simulink model "scalar_quantizer_example2"  (Simulink 5.0)
settings: Solver=FixedStepDiscrete  SolverMode=SingleTasking  StartTime=0.0  StopTime=0.49  RelTol=1e-3
PreLoadFcn:
  | load mtlb;
undefined symbols (not defined in the file or in its folder): Mag, mtlb
libraries: dspsnks4 x5, dspquant2 x5, dsparch4 x4, dspsigops x2, dspsrcs4 x1, dspstat3 x1, dspxfrm3 x1, dspsolvers x1, dspbuff3 x1
settings Model: RequirementInfo=9  CovMetricSettings=d  Creator=dshpak  LastModifiedBy=cclarke  ExtModeTrigMode=oneshot  ExtModeArmWhenConnect=off  ExtModeAutoUpdateStatusClock=off  SaveTime=off  SaveOutput=off  SaveFormat=Structure  LimitDataPoints=off  IntegerOverflowMsg=none  BlockReductionOpt=off  BooleanDataType=off  ZeroCrossControl=UseLocalSettings  TargetHWChar=2  TargetHWWordLengths=8,16,32,32  RTWMathFcnLibMatFile=iso_c_tmw.mat  RTWOptions="-aEnforceIntegerDowncast=1 -aFoldNonRolledExpr=1 -aInlineInvariantSignals=0 -aInlineParameters=0 -aLocalBlockOutputs=1 -aRollThreshold=5 -aRTWVerbose=1 -aForceParamTrailComments=0 -aGenerateComments=1 -aIgnoreCustomStorageClasses=1 -aIncHierarchyInIds=0 -aMaxRTWIdLen=31 -aShowEliminatedStatements=1 -aReadOnly=0 -aTargetFcnLib=\"iso_c_tmw.mat\" -aIncDataTypeInIds=0 -aPrefixModelToSubsysFcnNames=1 -aInlinedPrmAccess=\"Literals\" -aGenerateFullHeader=1 -aIsPILTarget=0 -aGenerateReport=0 -aLogVarNameModifier=\"rt_\" -aExtMode=0 -aExtModeStaticAlloc=0 -aExtModeTesting=0 -aExtModeStaticAllocSize=1000000 -aExtModeTransport=0"

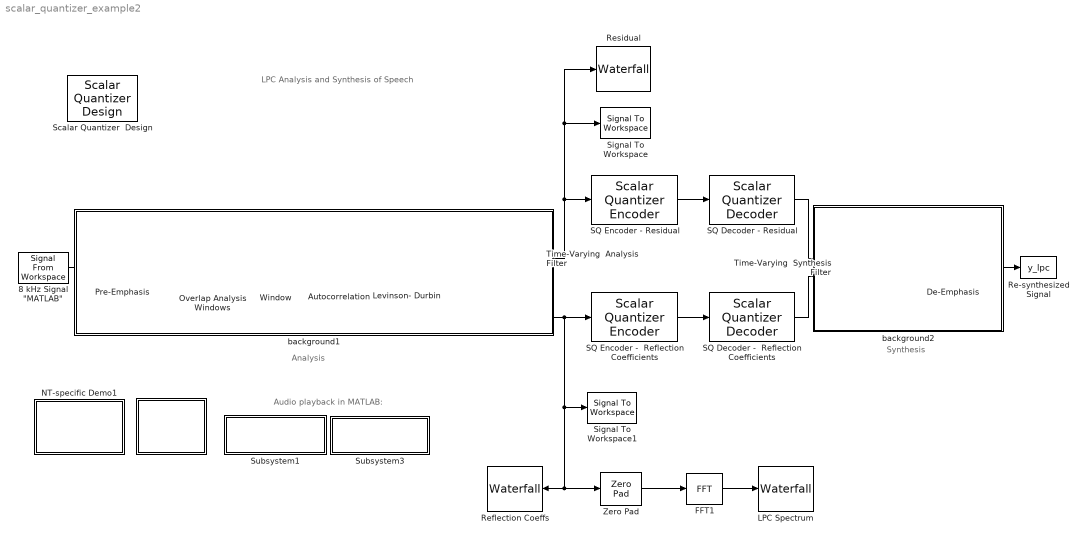
== system scalar_quantizer_example2 ==
  note: LPC Analysis and Synthesis of Speech
  note: Analysis
  note: Synthesis
  note: Audio playback in MATLAB:
  " " : Subsystem
      mask Type: Frame-Based Simulation Info
      mask Display: disp('Info')
  "8 kHz Signal \"MATLAB\"" : dspsrcs4/Signal From Workspace  X=mtlb*0.32  Ts=1/8000  nsamps=80  OutputAfterFinalValue=Setting to zero
  Autocorrelation : dspstat3/Autocorrelation  AllPositiveLags=off  maxlag=12  bias=Biased  domain=Time  roundingMode=Floor  overflowMode=off
  De-Emphasis : dsparch4/Digital Filter  TypePopup=IIR (all poles)  IIRFiltStruct=Direct form II transposed  AllPoleFiltStruct=Direct form  FIRFiltStruct=Direct form  CoeffSource=Specify via dialog  NumCoeffs=[1 -.95]  DenCoeffs=[1 -.95]  BiQuadCoeffs=[1 0.3 0.4 1 0.1 0.2]  LatticeCoeffs=[0.2 0.4]  denIgnore=on  FiltPerSampPopup=One filter per frame  IC=0  ICnum=0  ICden=0  roundingMode=Floor  overflowMode=off
  FFT1 : dspxfrm3/FFT  CompMethod=Table lookup  TableOpt=Speed  BitRevOrder=off  SkipNorm=off  roundingMode=Floor  overflowMode=off
  LPC Spectrum : dspsnks4/Waterfall  TraceProperties=off  NumTraces=10  CMapStr=autumn  TNewest=0.35  TOldest=0.1  HistoryLength=100  HistoryFull=Overwrite  UpdateInterval=1  ExportMode=All visible  MLExportName=ExportData  AutoExport=off  DisplayProperties=off  MouseMode=Orbit  AxisGrid=off  Snapshot=off  Suspend=off  SyncSnapshots=off  OpenScopeAtSimStart=off  FigPos=[452 44 407 353]  CameraView=[89945.9047576273 49093.2447020758 -7462.52930692949 -16.6995606364064 71 5.5 2.5389885178677 -5.30668596526891 0.808418434368868 0.0592442608385446 5.583225828012 14.2 1]  InportDimsHint=[129 1]  AxisProperties=off  AxisColor=[1 1 1]*.9  XLabel=Frequency  YLabel=Mag^2  ZLabel=History  TriggerProperties=off  TrigStartMode=Immediately  TrigStartT=10  TrigStartN=1000  TrigStartFcn=trigPower  TrigStopMode=Never  TrigStopT=0.1  TrigStopN=10  TrigStopFcn=trigend  TrigRearmMode=User-defined  TrigRearmT=0  TrigRearmN=100  TrigRearmFcn=trigrearm  XformProperties=off  XformMode=FFT->Mag dB Fs/2  XformFcn=fliplr  XformExpr=20*log10(abs(u(129:2:end)))
      settings: YMin=-44.6156897764664  YMax=11.2165685036536
  Levinson- Durbin : dspsolvers/Levinson-Durbin  coeffOutFcn=K  outP=off  zeroInpHandling=on
  NT-specific Demo1 : Subsystem
      settings: OpenFcn=dsplpc_win32
      mask Type: NT-only Demo
      mask Display: disp('PC/Windows\nLPC Demo')
  Overlap Analysis Windows : dspbuff3/Buffer  N=160  V=80  ic=0
  Pre-Emphasis : dsparch4/Digital Filter  TypePopup=FIR (all zeros)  IIRFiltStruct=Direct form II transposed  AllPoleFiltStruct=Direct form  FIRFiltStruct=Direct form  CoeffSource=Specify via dialog  NumCoeffs=[1 -.95]  DenCoeffs=[1 0.1]  BiQuadCoeffs=[1 0.3 0.4 1 0.1 0.2]  LatticeCoeffs=[0.2 0.4]  denIgnore=on  FiltPerSampPopup=One filter per frame  IC=0  ICnum=0  ICden=0  roundingMode=Floor  overflowMode=off
  Re-synthesized Signal : ToWorkspace  VariableName=y_lpc  SampleTime=-1  SaveFormat=Array
  Reflection Coeffs : dspsnks4/Waterfall  Orientation=left  TraceProperties=off  NumTraces=10  CMapStr=autumn  TNewest=0.7  TOldest=0.1  HistoryLength=50  HistoryFull=Overwrite  UpdateInterval=1  ExportMode=All visible  MLExportName=ExportData2  AutoExport=off  DisplayProperties=off  MouseMode=Orbit  AxisGrid=on  Snapshot=off  Suspend=off  SyncSnapshots=off  OpenScopeAtSimStart=off  FigPos=[35 41 410 358]  CameraView=[73343.0440471642 150383.489958622 -231607.055769344 -0.0735265549347769 7.5 5.5 0.547487828138618 -2.62241953831449 4.03911084299836 0.00240035045613671 1 7.88928028685195 5.25952019123463]  InportDimsHint=[12 1]  AxisProperties=off  AxisColor=[1 1 1]*.9  XLabel=Coefficient  YLabel=RC Amplitude  ZLabel=History  TriggerProperties=off  TrigStartMode=Immediately  TrigStartT=10  TrigStartN=1000  TrigStartFcn=trigPower  TrigStopMode=Never  TrigStopT=0.1  TrigStopN=10  TrigStopFcn=trigend  TrigRearmMode=User-defined  TrigRearmT=0  TrigRearmN=100  TrigRearmFcn=trigrearm  XformProperties=off  XformMode=None  XformFcn=fliplr  XformExpr=20*log10(abs(u(129:2:end)))
      settings: YMin=-1.02418361455266  YMax=0.877130504683106
  Residual : dspsnks4/Waterfall  TraceProperties=off  NumTraces=10  CMapStr=autumn  TNewest=0.7  TOldest=0.1  HistoryLength=50  HistoryFull=Overwrite  UpdateInterval=1  ExportMode=All visible  MLExportName=ExportData2  AutoExport=off  DisplayProperties=off  MouseMode=Orbit  AxisGrid=on  Snapshot=off  Suspend=off  SyncSnapshots=off  OpenScopeAtSimStart=off  FigPos=[524 276 410 358]  CameraView=[62164.2347969079 1792549.89917746 -405278.370332737 -0.097024155318337 44.5 5.5 0.575539043328793 -33.5051317778483 7.57548038023531 0.00104183380472551 1 92.0645761641202 10.3443344004629]  InportDimsHint=[80 1]  AxisProperties=off  AxisColor=[1 1 1]*.9  XLabel=Coefficient  YLabel=Amplitude  ZLabel=History  TriggerProperties=off  TrigStartMode=Immediately  TrigStartT=10  TrigStartN=1000  TrigStartFcn=trigPower  TrigStopMode=Never  TrigStopT=0.1  TrigStopN=10  TrigStopFcn=trigend  TrigRearmMode=User-defined  TrigRearmT=0  TrigRearmN=100  TrigRearmFcn=trigrearm  XformProperties=off  XformMode=None  XformFcn=fliplr  XformExpr=20*log10(abs(u(129:2:end)))
      settings: YMin=-0.580380532484202  YMax=0.386332221847528
  SQ Decoder -  Reflection Coefficients : dspquant2/Scalar Quantizer Decoder  Tag=SQDESIGN_GUI_REALIZE_MODEL  CBsource=Specify via dialog  codebook="[-0.93108    -0.91578    -0.90225    -0.85885    -0.84421     -0.8286    -0.81712    -0.78966    -0.76767    -0.74324    -0.72758    -0.71545    -0.62453    -0.59909    -0.58999    -0.56847    -0.56322    -0.54348    -0.51668    -0.50859    -0.49049     -0.4556     -0.4112    -0.40503    -0.39626    -0.37809    -0.36536    -0.36021    -0.35285    -0.34363     -0.3372     -0.3301    -0.32038    -0.31761    -0.29858    -0.29426    -0.29257    -0.28673    -0.27953    -0.27001    -0.25932    -0.24585    -0.23956    -0.23087    -0.22079    -0.21233    -0.20536    -0.20213    -0.19558    -0.18676    -0.18329    -0.17836    -0.16619    -0.15805    -0.14568    -0.13548    -0.12702    -0.12077    -0.10903   -0.099053   -0.093618   -0.087443   -0.079056   -0.069229   -0.059555   -0.046604   -0.033455    -0.01932  -0.0071711   0.0094043    0.022533    0.035599    0.051124    0.062732    0.076441    0.086143    0.098613     0.11395     0.13021     0.14046     0.15581     0.17205     0.18374     0.19465     0.20802     0.21992     0.23124     0.23747     0.24672     0.25728     0.26801     0.28141     0.29254     0.30396     0.31156     0.33072     0.34643     0.36327     0.37413     0.38123      0.3909     0.39705     0.40052     0.43217     0.44096     0.46456     0.48114     0.50022       0.508     0.51816     0.53742     0.54416     0.56371     0.57642     0.58657     0.60297       0.614     0.63125     0.63814     0.65711     0.66783     0.68146     0.69445     0.70759     0.75406      0.7643     0.77671     0.79739]"  invalidin=Clip  cwdtype=Double  outputMode=User-defined  outputWordLength=16  outputFracLength=15
      settings: allowOverrides=off
  SQ Decoder - Residual : dspquant2/Scalar Quantizer Decoder  Tag=SQDESIGN_GUI_REALIZE_MODEL  CBsource=Specify via dialog  codebook="[-0.52762    -0.50434    -0.48686    -0.48023    -0.47847      -0.471    -0.46439    -0.45511     -0.4483    -0.44149    -0.41351    -0.40777    -0.38649    -0.38257    -0.34459    -0.33656      -0.332    -0.31506     -0.3058    -0.29467    -0.28964    -0.27695    -0.26405    -0.25569    -0.24792    -0.24257    -0.23586    -0.22862     -0.2106    -0.20577    -0.20412    -0.18901    -0.18326    -0.17976    -0.17701    -0.17353    -0.16764    -0.16375    -0.15999    -0.15604    -0.15179    -0.14868    -0.14379    -0.13796    -0.13635    -0.13256    -0.13017    -0.12998    -0.12647    -0.12418    -0.11813     -0.1136    -0.11155    -0.11052    -0.10963    -0.10743    -0.10473    -0.10243     -0.1011   -0.099393   -0.096895   -0.094117   -0.089935   -0.085798   -0.081628   -0.076302   -0.068999   -0.061675   -0.053416   -0.045539   -0.039235   -0.031285   -0.023645   -0.016735   -0.011309  -0.0064137  -0.0017528   0.0031653   0.0083379    0.013857    0.020398      0.0273    0.035732    0.044282    0.051892    0.058205    0.064287    0.068767    0.072477     0.07818    0.082855    0.086893    0.093341     0.10139     0.10818     0.11338     0.12005      0.1266      0.1299     0.13376     0.13746     0.14153     0.14549     0.14866     0.14958     0.15164     0.15552     0.15703     0.15896     0.16211      0.1658     0.16848     0.17145     0.17815      0.1849      0.1891     0.19733     0.20475     0.20935     0.21575     0.22642     0.23266     0.23916     0.24329     0.25005      0.2589     0.27394     0.35121]"  invalidin=Clip  cwdtype=Double  outputMode=User-defined  outputWordLength=16  outputFracLength=15
      settings: allowOverrides=off
  SQ Encoder -  Reflection Coefficients : dspquant2/Scalar Quantizer Encoder  Tag=SQDESIGN_GUI_REALIZE_MODEL  paramSrc=Specify via dialog  partType=Bounded  BBoundary="[-inf -0.92343    -0.90902    -0.88055    -0.85153     -0.8364    -0.82286    -0.80339    -0.77867    -0.75545    -0.73541    -0.72151    -0.66999    -0.61181    -0.59454    -0.57923    -0.56585    -0.55335    -0.53008    -0.51263    -0.49954    -0.47304     -0.4334    -0.40811    -0.40064    -0.38717    -0.37172    -0.36279    -0.35653    -0.34824    -0.34041    -0.33365    -0.32524      -0.319    -0.30809    -0.29642    -0.29341    -0.28965    -0.28313    -0.27477    -0.26467    -0.25259    -0.24271    -0.23521    -0.22583    -0.21656    -0.20885    -0.20375    -0.19885    -0.19117    -0.18502    -0.18083    -0.17228    -0.16212    -0.15186    -0.14058    -0.13125     -0.1239     -0.1149    -0.10404   -0.096335    -0.09053    -0.08325   -0.074142   -0.064392    -0.05308    -0.04003   -0.026387   -0.013245   0.0011166    0.015969    0.029066    0.043362    0.056928    0.069587    0.081292    0.092378     0.10628     0.12208     0.13533     0.14814     0.16393      0.1779      0.1892     0.20133     0.21397     0.22558     0.23436     0.24209       0.252     0.26265     0.27471     0.28698     0.29825     0.30776     0.32114     0.33858     0.35485      0.3687     0.37768     0.38607     0.39397     0.39878     0.41634     0.43657     0.45276     0.47285     0.49068     0.50411     0.51308     0.52779     0.54079     0.55394     0.57007      0.5815     0.59477     0.60849     0.62263     0.63469     0.64762     0.66247     0.67464     0.68796     0.70102     0.73082     0.75918      0.7705     0.78705  +inf]"  UBoundary="[ -0.92343    -0.90902    -0.88055    -0.85153     -0.8364    -0.82286    -0.80339    -0.77867    -0.75545    -0.73541    -0.72151    -0.66999    -0.61181    -0.59454    -0.57923    -0.56585    -0.55335    -0.53008    -0.51263    -0.49954    -0.47304     -0.4334    -0.40811    -0.40064    -0.38717    -0.37172    -0.36279    -0.35653    -0.34824    -0.34041    -0.33365    -0.32524      -0.319    -0.30809    -0.29642    -0.29341    -0.28965    -0.28313    -0.27477    -0.26467    -0.25259    -0.24271    -0.23521    -0.22583    -0.21656    -0.20885    -0.20375    -0.19885    -0.19117    -0.18502    -0.18083    -0.17228    -0.16212    -0.15186    -0.14058    -0.13125     -0.1239     -0.1149    -0.10404   -0.096335    -0.09053    -0.08325   -0.074142   -0.064392    -0.05308    -0.04003   -0.026387   -0.013245   0.0011166    0.015969    0.029066    0.043362    0.056928    0.069587    0.081292    0.092378     0.10628     0.12208     0.13533     0.14814     0.16393      0.1779      0.1892     0.20133     0.21397     0.22558     0.23436     0.24209       0.252     0.26265     0.27471     0.28698     0.29825     0.30776     0.32114     0.33858     0.35485      0.3687     0.37768     0.38607     0.39397     0.39878     0.41634     0.43657     0.45276     0.47285     0.49068     0.50411     0.51308     0.52779     0.54079     0.55394     0.57007      0.5815     0.59477     0.60849     0.62263     0.63469     0.64762     0.66247     0.67464     0.68796     0.70102     0.73082     0.75918      0.7705     0.78705  ]"  SearchMethod=Binary  tieBreakRule=Choose the lower index  outQU=off  outQError=off  codebook="[-0.93108    -0.91578    -0.90225    -0.85885    -0.84421     -0.8286    -0.81712    -0.78966    -0.76767    -0.74324    -0.72758    -0.71545    -0.62453    -0.59909    -0.58999    -0.56847    -0.56322    -0.54348    -0.51668    -0.50859    -0.49049     -0.4556     -0.4112    -0.40503    -0.39626    -0.37809    -0.36536    -0.36021    -0.35285    -0.34363     -0.3372     -0.3301    -0.32038    -0.31761    -0.29858    -0.29426    -0.29257    -0.28673    -0.27953    -0.27001    -0.25932    -0.24585    -0.23956    -0.23087    -0.22079    -0.21233    -0.20536    -0.20213    -0.19558    -0.18676    -0.18329    -0.17836    -0.16619    -0.15805    -0.14568    -0.13548    -0.12702    -0.12077    -0.10903   -0.099053   -0.093618   -0.087443   -0.079056   -0.069229   -0.059555   -0.046604   -0.033455    -0.01932  -0.0071711   0.0094043    0.022533    0.035599    0.051124    0.062732    0.076441    0.086143    0.098613     0.11395     0.13021     0.14046     0.15581     0.17205     0.18374     0.19465     0.20802     0.21992     0.23124     0.23747     0.24672     0.25728     0.26801     0.28141     0.29254     0.30396     0.31156     0.33072     0.34643     0.36327     0.37413     0.38123      0.3909     0.39705     0.40052     0.43217     0.44096     0.46456     0.48114     0.50022       0.508     0.51816     0.53742     0.54416     0.56371     0.57642     0.58657     0.60297       0.614     0.63125     0.63814     0.65711     0.66783     0.68146     0.69445     0.70759     0.75406      0.7643     0.77671     0.79739]"  outStatus=off  invalidin=Clip  idtype=int32  roundingMode=Nearest  overflowMode=on
  SQ Encoder - Residual : dspquant2/Scalar Quantizer Encoder  Tag=SQDESIGN_GUI_REALIZE_MODEL  paramSrc=Specify via dialog  partType=Bounded  BBoundary="[-inf -0.51598     -0.4956    -0.48355    -0.47935    -0.47473    -0.46769    -0.45975     -0.4517     -0.4449     -0.4275    -0.41064    -0.39713    -0.38453    -0.36358    -0.34057    -0.33428    -0.32353    -0.31043    -0.30024    -0.29216    -0.28329     -0.2705    -0.25987     -0.2518    -0.24524    -0.23922    -0.23224    -0.21961    -0.20819    -0.20495    -0.19656    -0.18613    -0.18151    -0.17839    -0.17527    -0.17058    -0.16569    -0.16187    -0.15802    -0.15392    -0.15024    -0.14624    -0.14088    -0.13716    -0.13446    -0.13136    -0.13007    -0.12823    -0.12533    -0.12115    -0.11587    -0.11258    -0.11103    -0.11007    -0.10853    -0.10608    -0.10358    -0.10176    -0.10024   -0.098144   -0.095506   -0.092026   -0.087867   -0.083713   -0.078965   -0.072651   -0.065337   -0.057545   -0.049477   -0.042387    -0.03526   -0.027465    -0.02019   -0.014022  -0.0088614  -0.0040832  0.00070626   0.0057516    0.011097    0.017127    0.023849    0.031516    0.040007    0.048087    0.055049    0.061246    0.066527    0.070622    0.075328    0.080518    0.084874    0.090117    0.097368     0.10479     0.11078     0.11671     0.12332     0.12825     0.13183     0.13561      0.1395     0.14351     0.14707     0.14912     0.15061     0.15358     0.15628       0.158     0.16054     0.16396     0.16714     0.16996      0.1748     0.18152       0.187     0.19321     0.20104     0.20705     0.21255     0.22109     0.22954     0.23591     0.24122     0.24667     0.25447     0.26642     0.31258  +inf]"  UBoundary="[ -0.51598     -0.4956    -0.48355    -0.47935    -0.47473    -0.46769    -0.45975     -0.4517     -0.4449     -0.4275    -0.41064    -0.39713    -0.38453    -0.36358    -0.34057    -0.33428    -0.32353    -0.31043    -0.30024    -0.29216    -0.28329     -0.2705    -0.25987     -0.2518    -0.24524    -0.23922    -0.23224    -0.21961    -0.20819    -0.20495    -0.19656    -0.18613    -0.18151    -0.17839    -0.17527    -0.17058    -0.16569    -0.16187    -0.15802    -0.15392    -0.15024    -0.14624    -0.14088    -0.13716    -0.13446    -0.13136    -0.13007    -0.12823    -0.12533    -0.12115    -0.11587    -0.11258    -0.11103    -0.11007    -0.10853    -0.10608    -0.10358    -0.10176    -0.10024   -0.098144   -0.095506   -0.092026   -0.087867   -0.083713   -0.078965   -0.072651   -0.065337   -0.057545   -0.049477   -0.042387    -0.03526   -0.027465    -0.02019   -0.014022  -0.0088614  -0.0040832  0.00070626   0.0057516    0.011097    0.017127    0.023849    0.031516    0.040007    0.048087    0.055049    0.061246    0.066527    0.070622    0.075328    0.080518    0.084874    0.090117    0.097368     0.10479     0.11078     0.11671     0.12332     0.12825     0.13183     0.13561      0.1395     0.14351     0.14707     0.14912     0.15061     0.15358     0.15628       0.158     0.16054     0.16396     0.16714     0.16996      0.1748     0.18152       0.187     0.19321     0.20104     0.20705     0.21255     0.22109     0.22954     0.23591     0.24122     0.24667     0.25447     0.26642     0.31258  ]"  SearchMethod=Binary  tieBreakRule=Choose the lower index  outQU=off  outQError=off  codebook="[-0.52762    -0.50434    -0.48686    -0.48023    -0.47847      -0.471    -0.46439    -0.45511     -0.4483    -0.44149    -0.41351    -0.40777    -0.38649    -0.38257    -0.34459    -0.33656      -0.332    -0.31506     -0.3058    -0.29467    -0.28964    -0.27695    -0.26405    -0.25569    -0.24792    -0.24257    -0.23586    -0.22862     -0.2106    -0.20577    -0.20412    -0.18901    -0.18326    -0.17976    -0.17701    -0.17353    -0.16764    -0.16375    -0.15999    -0.15604    -0.15179    -0.14868    -0.14379    -0.13796    -0.13635    -0.13256    -0.13017    -0.12998    -0.12647    -0.12418    -0.11813     -0.1136    -0.11155    -0.11052    -0.10963    -0.10743    -0.10473    -0.10243     -0.1011   -0.099393   -0.096895   -0.094117   -0.089935   -0.085798   -0.081628   -0.076302   -0.068999   -0.061675   -0.053416   -0.045539   -0.039235   -0.031285   -0.023645   -0.016735   -0.011309  -0.0064137  -0.0017528   0.0031653   0.0083379    0.013857    0.020398      0.0273    0.035732    0.044282    0.051892    0.058205    0.064287    0.068767    0.072477     0.07818    0.082855    0.086893    0.093341     0.10139     0.10818     0.11338     0.12005      0.1266      0.1299     0.13376     0.13746     0.14153     0.14549     0.14866     0.14958     0.15164     0.15552     0.15703     0.15896     0.16211      0.1658     0.16848     0.17145     0.17815      0.1849      0.1891     0.19733     0.20475     0.20935     0.21575     0.22642     0.23266     0.23916     0.24329     0.25005      0.2589     0.27394     0.35121]"  outStatus=off  invalidin=Clip  idtype=int32  roundingMode=Nearest  overflowMode=on
  Scalar Quantizer  Design : dspquant2/Scalar Quantizer  Design
  Signal To Workspace : dspsnks4/Signal To Workspace  VariableName=E  FrameMode=Concatenate frames (2-D array)
  Signal To Workspace1 : dspsnks4/Signal To Workspace  VariableName=K  FrameMode=Concatenate frames (2-D array)
  Subsystem1 : Subsystem
      settings: OpenFcn=if exist('mtlb','var'), sound(mtlb*0.32,8000); else errordlg('Data not found in workspace - reload demo model.','DSP Blockset Demo Error'); end
      mask Display: disp('Original\nSignal')
  Subsystem3 : Subsystem
      settings: OpenFcn=if exist('y_lpc','var'), sound(y_lpc,8000); else errordlg('You must run the simulation first.','DSP Blockset Demo Error'); end
      mask Display: disp('Processed\nSignal')
  Time-Varying  Analysis Filter : dsparch4/Digital Filter  TypePopup=FIR (all zeros)  IIRFiltStruct=Direct form II transposed  AllPoleFiltStruct=Direct form  FIRFiltStruct=Lattice MA  CoeffSource=Input port(s)  NumCoeffs=[1 -.95]  DenCoeffs=[1 0.1]  BiQuadCoeffs=[1 0.3 0.4 1 0.1 0.2]  LatticeCoeffs=[0.2 0.4]  denIgnore=on  FiltPerSampPopup=One filter per frame  IC=0  ICnum=0  ICden=0  roundingMode=Floor  overflowMode=off
  Time-Varying  Synthesis Filter : dsparch4/Digital Filter  TypePopup=IIR (all poles)  IIRFiltStruct=Direct form II transposed  AllPoleFiltStruct=Lattice AR  FIRFiltStruct=Direct form  CoeffSource=Input port(s)  NumCoeffs=[1 -.95]  DenCoeffs=[1 0.1]  BiQuadCoeffs=[1 0.3 0.4 1 0.1 0.2]  LatticeCoeffs=[0.2 0.4]  denIgnore=on  FiltPerSampPopup=One filter per frame  IC=0  ICnum=0  ICden=0  roundingMode=Floor  overflowMode=off
  Window : dspsigops/Window Function  winmode=Apply window to input  wintype=Hamming  sampmode=Continuous  samptime=1  N=64  Rs=50  beta=10  winsamp=Symmetric  UserWindow=hamming  OptParams=off  UserParams={1.0}  dataType=double  wordLen=16  udDataType=sfix(16)  fracBitsMode=Best precision  numFracBits=15  roundingMode=Floor  overflowMode=off
  Zero Pad : dspsigops/Zero Pad  padSigAt=End  zpadAlong=Columns  padNumOutRowsSpecMethod=User-specified  numOutRows=256  padNumOutColsSpecMethod=User-specified  numOutCols=1  trunc_flag=None
  background1 : Subsystem
      mask Display: disp('')
  background2 : Subsystem
      mask Display: disp('')
  wires:
  "8 kHz Signal \"MATLAB\""/1 -> Pre-Emphasis/1
  Pre-Emphasis/1 -> Overlap Analysis Windows/1, Time-Varying  Analysis Filter/1
  Overlap Analysis Windows/1 -> Window/1
  Autocorrelation/1 -> Levinson- Durbin/1
  Window/1 -> Autocorrelation/1
  Time-Varying  Analysis Filter/1 -> Residual/1, Signal To Workspace/1, SQ Encoder - Residual/1
  Levinson- Durbin/1 -> Time-Varying  Analysis Filter/2, Reflection Coeffs/1, Zero Pad/1, Signal To Workspace1/1, SQ Encoder -  Reflection Coefficients/1
  Time-Varying  Synthesis Filter/1 -> De-Emphasis/1
  De-Emphasis/1 -> Re-synthesized Signal/1
  Zero Pad/1 -> FFT1/1
  FFT1/1 -> LPC Spectrum/1
  SQ Encoder -  Reflection Coefficients/1 -> SQ Decoder -  Reflection Coefficients/1
  SQ Encoder - Residual/1 -> SQ Decoder - Residual/1
  SQ Decoder - Residual/1 -> Time-Varying  Synthesis Filter/1
  SQ Decoder -  Reflection Coefficients/1 -> Time-Varying  Synthesis Filter/2

== system scalar_quantizer_example2/  ==
  note: LPC Analysis and Synthesis of Speech
      |
      | This demo consists of two parts,  analysis and synthesis. The analysis part
      | is found in the transmitter section of a system. Using the original speech signal, parameters
      | (reflection coefficients) and the residual signal are extracted from it, and then transmitted over
      | a channel. The synthesis part , which is found in the receiver section of the system, reconstructs
      | the original signal using those parameters and the residual signal.
      |
      | In this simulation , the speech signal is divided into
      | frames of size 20 ms (160 samples) , with an overlap of 10 ms (80 samples).Each frame
      | is then windowed using a hamming window, 11th order autocorrelation coefficients
      | are found and then the reflection coefficients (11th order) are calculated from the autocorrelation
      | coefficients, using the Levinson-Durbin algorithm. The original speech signal is passed through an
      |  analysis-filter which is basically an all-zero filter with coefficients as the reflection coefficients
      | obtained above. The output of the filter is the residual signal. This residual signal is then
      | passed through a synthesis-filter which is basically an all-pole filter, again with coefficients as the
      | reflection coefficients (Synthesis filter is just the inverse of Analysis filter). The output of the
      | synthesis filter is the original signal.

== system scalar_quantizer_example2/NT-specific Demo1 ==

== system scalar_quantizer_example2/Subsystem1 ==

== system scalar_quantizer_example2/Subsystem3 ==

== system scalar_quantizer_example2/background1 ==

== system scalar_quantizer_example2/background2 ==
